simulink model "L2_s"  (R2023a)
settings: Solver=FixedStepAuto  StartTime=0.0  StopTime=70  FixedStep=1e-4  RelTol=1e-6
InitFcn:
  | l = 2.5;
  | m = 0.75;
  | c = 0.15;
  | g = 9.81;
settings Model: Creator=LabCom  LastModifiedBy=LabCom

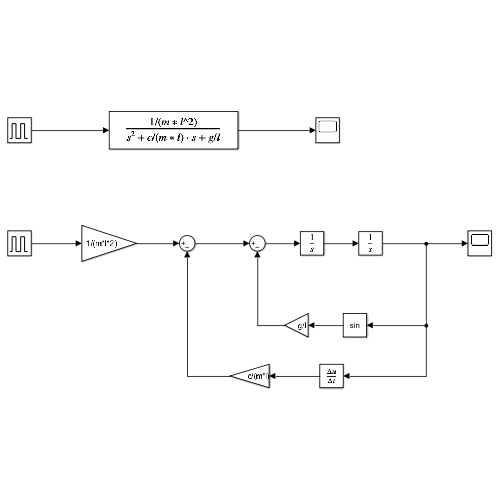
[thumbnail: Simulink's stored preview of the top-level diagram]
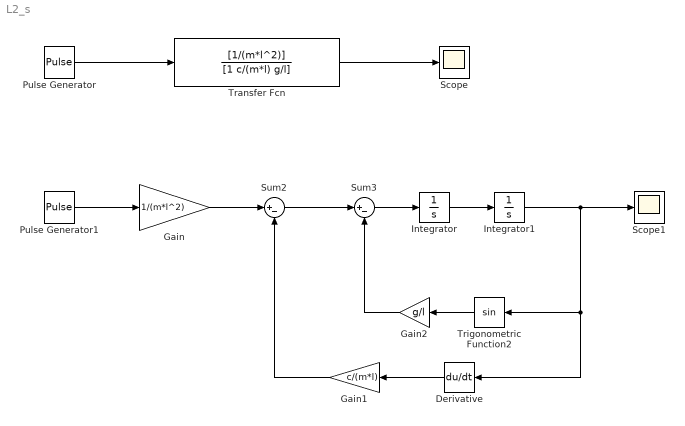
== system L2_s ==
  Derivative : Derivative
  Gain : Gain  Gain=1/(m*l^2)
  Gain1 : Gain  Gain=c/(m*l)
  Gain2 : Gain  Gain=g/l
  Integrator : Integrator
  Integrator1 : Integrator
  Pulse Generator : DiscretePulseGenerator  PulseType=Time based  Amplitude=20  Period=100  PulseWidth=0.1
  Pulse Generator1 : DiscretePulseGenerator  PulseType=Time based  Amplitude=20  Period=100  PulseWidth=0.1
  Scope : Scope
  Scope1 : Scope
  Sum2 : Sum  Inputs=|+-
  Sum3 : Sum  Inputs=|+-
  Transfer Fcn : TransferFcn  Numerator=[1/(m*l^2)]  Denominator=[1 c/(m*l) g/l]
  Trigonometric Function2 : Trigonometry
  wires:
  Pulse Generator/1 -> Transfer Fcn/1
  Transfer Fcn/1 -> Scope/1
  Pulse Generator1/1 -> Gain/1
  Gain1/1 -> Sum2/2
  Gain/1 -> Sum2/1
  Sum2/1 -> Sum3/1
  Derivative/1 -> Gain1/1
  Gain2/1 -> Sum3/2
  Sum3/1 -> Integrator/1
  Integrator1/1 -> Scope1/1, Trigonometric Function2/1, Derivative/1
  Trigonometric Function2/1 -> Gain2/1
  Integrator/1 -> Integrator1/1
